simulink model "c6_pfc_rl"  (R2021b)
settings: Solver=FixedStepDiscrete  StartTime=0.0  StopTime=Inf  FixedStep=sampleTime  RelTol=1e-3  EnableMultiTasking=on
PreLoadFcn:
  | %load emptyMap
InitFcn:
  | sampleTime = 0.05;
  | nMedianSize=3;
  | 
  | % Robot parameters
  | wheelRadius = 0.0335;
  | robotRadius = 0.116;
  | 
  | % Lidar parameters
  | sensorOffset = [0,0];
  | scanAngles = linspace(-pi/2,pi/2,9)';
  | maxRange = 5;
  | 
  | %%%%%%
  | ks=1;
  | c_ks=-1;
  | 
  | 
  | 
  | 
  | 
  | 
  | % Lidar parameters
  | sensorOffset = [0,0];
  | scanAngles = linspace(-pi/3,pi/3,20)';%y = linspace(x1,x2,n) 生成 n 个点。这些点的间距为 (x2-x1)/(n-1)。
  | maxRange = 0.4;
  | 
  | %%%%%%
  | ks=1;
  | 
  | 
  | 
  | 
  | 
  | A=0.3;
  | C=1.7;
  | B=(A+C)/2;
  | 
  | wp1=[A,A; B,A;  C,A; C,B;C,C; B,C; A,C;A,B];
  | bainjie2=[-0.5,-0.5;2.5,-0.5;-0.5,2.5;2.5,2.5;]
  | WAY_P=[wp1;wp1;wp1;wp1];
  | Target=[wp1;bainjie2];
  | 
  | %%%%%%%%%%%%%%%%%%%%%%%%%%%%%%%%%%%%%%%
  | Target_robot_4=[A  A]
  | Target_robot_5=[B  A]
  | Target_robot_6=[C  A]
  | 
  | Target_robot_1=[C  C]
  | Target_robot_2=[B  C]
  | Target_robot_3=[A  C]
  | 
  | 
  | %%%%%%%%%%%%%%%%%%%%%%%%%%%%%%%%%%%%
  | 
  | 
  | 
  | 
  | 
  | % paremeters of pure persuit
  | desired_v_robot_1=0.2
  | ... (+33 lines)
undefined symbols (not defined in the file or in its folder): Angular, DiscIntNeverNeededParam, Linear
libraries: robotlib x24, dspstat3 x18, simulink x2, robotalgslib x1
(part 2 of 2)

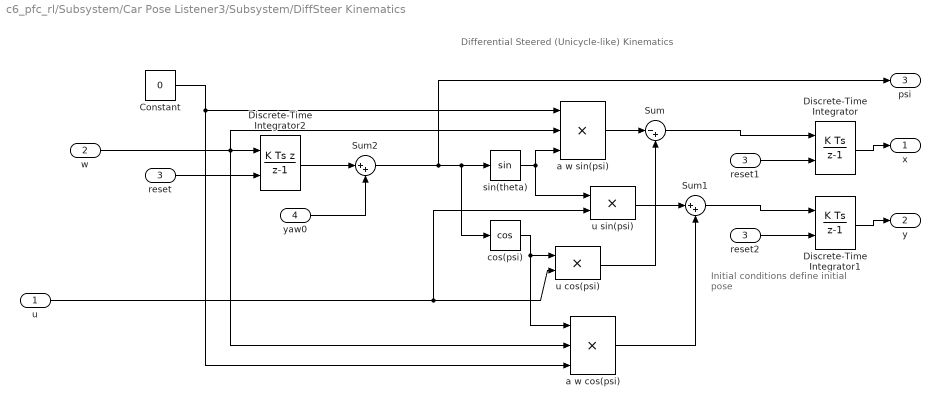
== system c6_pfc_rl/Subsystem/Car Pose Listener3/Subsystem/DiffSteer Kinematics ==
  note: Initial conditions define
      | initial pose
  note: Differential Steered (Unicycle-like) Kinematics
  u : Inport
  w : Inport  Port=2
  reset : Inport  Port=3
  yaw0 : Inport  Port=4
  Constant : Constant  Value=0
  Discrete-Time Integrator : DiscreteIntegrator  ExternalReset=falling  SampleTime=-1  ICPrevOutput=DiscIntNeverNeededParam  ICPrevScaledInput=DiscIntNeverNeededParam
  Discrete-Time Integrator1 : DiscreteIntegrator  ExternalReset=falling  SampleTime=-1  ICPrevOutput=DiscIntNeverNeededParam  ICPrevScaledInput=DiscIntNeverNeededParam
  Discrete-Time Integrator2 : DiscreteIntegrator  IntegratorMethod=Integration: Backward Euler  ExternalReset=falling  SampleTime=-1  ICPrevOutput=DiscIntNeverNeededParam  ICPrevScaledInput=DiscIntNeverNeededParam
  Sum : Sum  Inputs=|-+  SaturateOnIntegerOverflow=on
  Sum1 : Sum  Inputs=|++  SaturateOnIntegerOverflow=on
  Sum2 : Sum  Inputs=|++
  a w cos(psi) : Product  Inputs=3  SaturateOnIntegerOverflow=on  OutDataTypeStr=Inherit: Same as first input
  a w sin(psi) : Product  Inputs=3  SaturateOnIntegerOverflow=on  OutDataTypeStr=Inherit: Same as first input
  cos(psi) : Trigonometry  Operator=cos
  reset1 : InportShadow  Port=3
  reset2 : InportShadow  Port=3
  sin(theta) : Trigonometry
  u cos(psi) : Product  SaturateOnIntegerOverflow=on  OutDataTypeStr=Inherit: Same as first input
  u sin(psi) : Product  SaturateOnIntegerOverflow=on  OutDataTypeStr=Inherit: Same as first input
  x : Outport
  y : Outport  Port=2
  psi : Outport  Port=3
  wires:
  yaw0/1 -> Sum2/2
  reset2/1 -> Discrete-Time Integrator1/2
  reset1/1 -> Discrete-Time Integrator/2
  reset/1 -> Discrete-Time Integrator2/2
  u sin(psi)/1 -> Sum1/1
  cos(psi)/1 -> u cos(psi)/1, a w cos(psi)/1
  w/1 -> a w cos(psi)/2, a w sin(psi)/2, Discrete-Time Integrator2/1
  Constant/1 -> a w sin(psi)/1, a w cos(psi)/3
  Discrete-Time Integrator/1 -> x/1
  Sum/1 -> Discrete-Time Integrator/1
  sin(theta)/1 -> a w sin(psi)/3, u sin(psi)/1
  a w cos(psi)/1 -> Sum1/2
  Sum2/1 -> psi/1, sin(theta)/1, cos(psi)/1
  u cos(psi)/1 -> Sum/2
  u/1 -> u sin(psi)/2, u cos(psi)/2
  a w sin(psi)/1 -> Sum/1
  Sum1/1 -> Discrete-Time Integrator1/1
  Discrete-Time Integrator1/1 -> y/1
  Discrete-Time Integrator2/1 -> Sum2/1

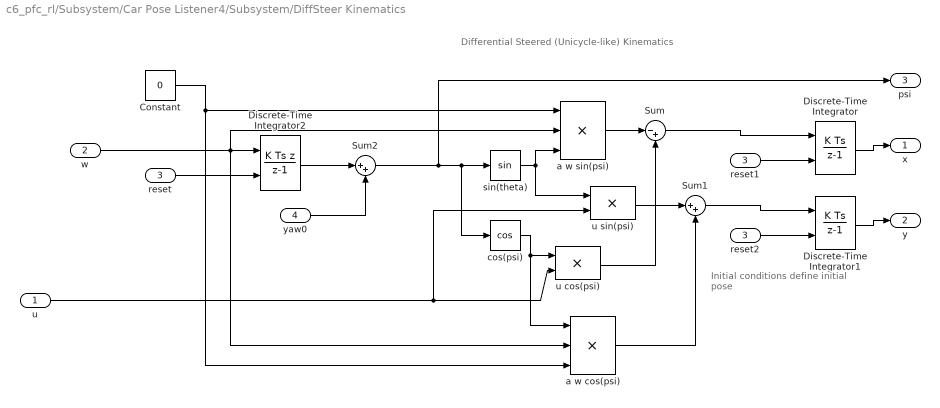
== system c6_pfc_rl/Subsystem/Car Pose Listener4/Subsystem/DiffSteer Kinematics ==
  note: Initial conditions define
      | initial pose
  note: Differential Steered (Unicycle-like) Kinematics
  u : Inport
  w : Inport  Port=2
  reset : Inport  Port=3
  yaw0 : Inport  Port=4
  Constant : Constant  Value=0
  Discrete-Time Integrator : DiscreteIntegrator  ExternalReset=falling  SampleTime=-1  ICPrevOutput=DiscIntNeverNeededParam  ICPrevScaledInput=DiscIntNeverNeededParam
  Discrete-Time Integrator1 : DiscreteIntegrator  ExternalReset=falling  SampleTime=-1  ICPrevOutput=DiscIntNeverNeededParam  ICPrevScaledInput=DiscIntNeverNeededParam
  Discrete-Time Integrator2 : DiscreteIntegrator  IntegratorMethod=Integration: Backward Euler  ExternalReset=falling  SampleTime=-1  ICPrevOutput=DiscIntNeverNeededParam  ICPrevScaledInput=DiscIntNeverNeededParam
  Sum : Sum  Inputs=|-+  SaturateOnIntegerOverflow=on
  Sum1 : Sum  Inputs=|++  SaturateOnIntegerOverflow=on
  Sum2 : Sum  Inputs=|++
  a w cos(psi) : Product  Inputs=3  SaturateOnIntegerOverflow=on  OutDataTypeStr=Inherit: Same as first input
  a w sin(psi) : Product  Inputs=3  SaturateOnIntegerOverflow=on  OutDataTypeStr=Inherit: Same as first input
  cos(psi) : Trigonometry  Operator=cos
  reset1 : InportShadow  Port=3
  reset2 : InportShadow  Port=3
  sin(theta) : Trigonometry
  u cos(psi) : Product  SaturateOnIntegerOverflow=on  OutDataTypeStr=Inherit: Same as first input
  u sin(psi) : Product  SaturateOnIntegerOverflow=on  OutDataTypeStr=Inherit: Same as first input
  x : Outport
  y : Outport  Port=2
  psi : Outport  Port=3
  wires:
  yaw0/1 -> Sum2/2
  reset2/1 -> Discrete-Time Integrator1/2
  reset1/1 -> Discrete-Time Integrator/2
  reset/1 -> Discrete-Time Integrator2/2
  u sin(psi)/1 -> Sum1/1
  cos(psi)/1 -> u cos(psi)/1, a w cos(psi)/1
  w/1 -> a w cos(psi)/2, a w sin(psi)/2, Discrete-Time Integrator2/1
  Constant/1 -> a w sin(psi)/1, a w cos(psi)/3
  Discrete-Time Integrator/1 -> x/1
  Sum/1 -> Discrete-Time Integrator/1
  sin(theta)/1 -> a w sin(psi)/3, u sin(psi)/1
  a w cos(psi)/1 -> Sum1/2
  Sum2/1 -> psi/1, sin(theta)/1, cos(psi)/1
  u cos(psi)/1 -> Sum/2
  u/1 -> u sin(psi)/2, u cos(psi)/2
  a w sin(psi)/1 -> Sum/1
  Sum1/1 -> Discrete-Time Integrator1/1
  Discrete-Time Integrator1/1 -> y/1
  Discrete-Time Integrator2/1 -> Sum2/1

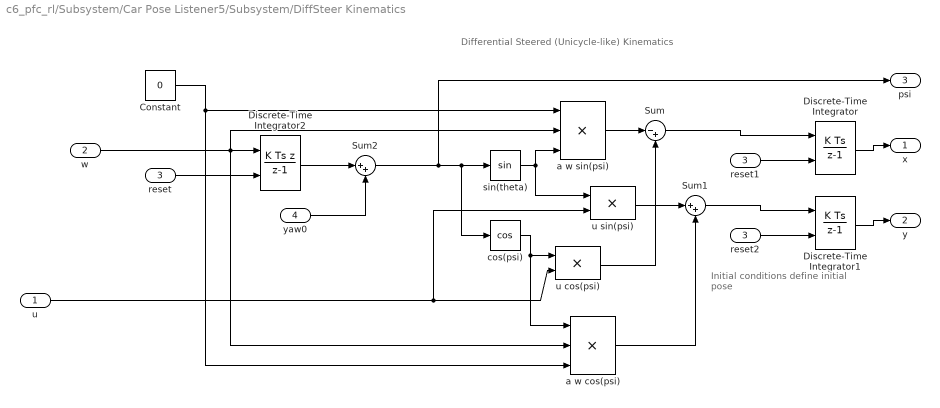
== system c6_pfc_rl/Subsystem/Car Pose Listener5/Subsystem/DiffSteer Kinematics ==
  note: Initial conditions define
      | initial pose
  note: Differential Steered (Unicycle-like) Kinematics
  u : Inport
  w : Inport  Port=2
  reset : Inport  Port=3
  yaw0 : Inport  Port=4
  Constant : Constant  Value=0
  Discrete-Time Integrator : DiscreteIntegrator  ExternalReset=falling  SampleTime=-1  ICPrevOutput=DiscIntNeverNeededParam  ICPrevScaledInput=DiscIntNeverNeededParam
  Discrete-Time Integrator1 : DiscreteIntegrator  ExternalReset=falling  SampleTime=-1  ICPrevOutput=DiscIntNeverNeededParam  ICPrevScaledInput=DiscIntNeverNeededParam
  Discrete-Time Integrator2 : DiscreteIntegrator  IntegratorMethod=Integration: Backward Euler  ExternalReset=falling  SampleTime=-1  ICPrevOutput=DiscIntNeverNeededParam  ICPrevScaledInput=DiscIntNeverNeededParam
  Sum : Sum  Inputs=|-+  SaturateOnIntegerOverflow=on
  Sum1 : Sum  Inputs=|++  SaturateOnIntegerOverflow=on
  Sum2 : Sum  Inputs=|++
  a w cos(psi) : Product  Inputs=3  SaturateOnIntegerOverflow=on  OutDataTypeStr=Inherit: Same as first input
  a w sin(psi) : Product  Inputs=3  SaturateOnIntegerOverflow=on  OutDataTypeStr=Inherit: Same as first input
  cos(psi) : Trigonometry  Operator=cos
  reset1 : InportShadow  Port=3
  reset2 : InportShadow  Port=3
  sin(theta) : Trigonometry
  u cos(psi) : Product  SaturateOnIntegerOverflow=on  OutDataTypeStr=Inherit: Same as first input
  u sin(psi) : Product  SaturateOnIntegerOverflow=on  OutDataTypeStr=Inherit: Same as first input
  x : Outport
  y : Outport  Port=2
  psi : Outport  Port=3
  wires:
  yaw0/1 -> Sum2/2
  reset2/1 -> Discrete-Time Integrator1/2
  reset1/1 -> Discrete-Time Integrator/2
  reset/1 -> Discrete-Time Integrator2/2
  u sin(psi)/1 -> Sum1/1
  cos(psi)/1 -> u cos(psi)/1, a w cos(psi)/1
  w/1 -> a w cos(psi)/2, a w sin(psi)/2, Discrete-Time Integrator2/1
  Constant/1 -> a w sin(psi)/1, a w cos(psi)/3
  Discrete-Time Integrator/1 -> x/1
  Sum/1 -> Discrete-Time Integrator/1
  sin(theta)/1 -> a w sin(psi)/3, u sin(psi)/1
  a w cos(psi)/1 -> Sum1/2
  Sum2/1 -> psi/1, sin(theta)/1, cos(psi)/1
  u cos(psi)/1 -> Sum/2
  u/1 -> u sin(psi)/2, u cos(psi)/2
  a w sin(psi)/1 -> Sum/1
  Sum1/1 -> Discrete-Time Integrator1/1
  Discrete-Time Integrator1/1 -> y/1
  Discrete-Time Integrator2/1 -> Sum2/1

== system c6_pfc_rl/controller/Subsystem1/Adjust Velocities to Avoid Obstacles/Path Following ==
  SteeringDirection : Inport
  AngularVelocity : Inport  Port=2
  Compute Angular Velocity : MATLAB Function  TreatAsAtomicUnit=on
  MaxAngularVelocity : Constant
  Subtract : Sum  Inputs=+-
  dW : Outport  VectorParamsAs1DForOutWhenUnconnected=off
  wires:
  MaxAngularVelocity/1 -> Compute Angular Velocity/2(wMax)
  SteeringDirection/1 -> Compute Angular Velocity/1(steeringDir)
  Subtract/1 -> dW/1
  Compute Angular Velocity/1(w) -> Subtract/1
  AngularVelocity/1 -> Subtract/2

== matlab function c6_pfc_rl/Subsystem/Car Pose Listener1/Subsystem/sensor2vCar ==
  data: x_init output; y_init output; yaw_init output; flag output; poseNew input; poseMsg input
function [x_init,y_init,yaw_init,flag] = sensor2vCar(poseNew, poseMsg)
persistent x0 y0 yaw0 yaw1 x0_init y0_init yaw0_init fStart
if isempty(x0)
    x0=-10; y0=-10; yaw0=0; yaw1=0;   
    x0_init=-10;y0_init=-10;yaw0_init=0;
    fStart=0;
end
if poseNew
    if x0==poseMsg.Pose.Pose.Position.X&&y0==poseMsg.Pose.Pose.Position.Y
        flag=1;
    else
        x0=poseMsg.Pose.Pose.Position.X;
        y0=poseMsg.Pose.Pose.Position.Y;   
        %yaw2=atan2(2*(poseMsg.Pose.Pose.Orientation.Z*poseMsg.Pose.Pose.Orientation.W),1-2*(poseMsg.Pose.Pose.Orientation.Z^2)); 
        eul=quat2eul([poseMsg.Pose.Pose.Orientation.W,poseMsg.Pose.Pose.Orientation.X,poseMsg.Pose.Pose.Orientation.Y,poseMsg.Pose.Pose.Orientation.Z]);
        yaw2=eul(1);
        %对前后角度差使用积分，恢复yaw的连续性
        yaw0=yaw0+angdiff(yaw1,yaw2);
        yaw1=yaw2;
        flag=0;        
        x0_init=x0;
        y0_init=y0;
        yaw0_init=yaw0;
        fStart=1;
    end 
else
    if fStart
        flag=1;
    else
        flag=0;
    end
end

x_init=x0_init;y_init=y0_init;yaw_init=yaw0_init;

== matlab function c6_pfc_rl/controller/MATLAB Function4 ==
  data: z output; pos1 input
function z = plot_a_square(pos1)
% 
% persistent Waypoints idx
% if isempty(Waypoints)
%     Waypoints=[0.2,0.2;1.8 0.2;1.8 1.8;0.2 1.8];
%     idx=0;
% end
% if idx==0
%     %初始化
%     [~,idx]=max([norm(Waypoints(1,:)-pos1(1:2)'),norm(Waypoints(2,:)-pos1(1:2)'),norm(Waypoints(3,:)-pos1(1:2)'),norm(Waypoints(4,:)-pos1(1:2)')]);
% end
% 
% if norm([Waypoints(idx,:)-pos1(1:2)'])<0.25
%     idx=idx+1;
%     if idx>length(Waypoints(:,1))
%         idx=1;
%     end
% end
% z=Waypoints(idx,:);


persistent Waypoints idx

if isempty(Waypoints)
    Waypoints=[0.5,0.5;1.5 0.5;1.5 1.5;0.5 1.5];
    idx=2;
end

if idx == 4
    pre_waypt = Waypoints(4-1,:)';
    curr_waypt = Waypoints(idx,:)';
    next_waypt = Waypoints(1,:)';
else
    if idx == 1
        pre_waypt = Waypoints(4,:)';
        curr_waypt = Waypoints(1,:)';
        next_waypt = Waypoints(2,:)';
    else
        pre_waypt = Waypoints(idx-1,:)';
        curr_waypt = Waypoints(idx,:)';
        next_waypt = Waypoints(idx+1,:)';
    end
end

pre_q = vec_norm(curr_waypt, pre_waypt);
next_q = vec_norm(next_waypt, curr_waypt);

curr_n = vec_normalize(pre_q + next_q);
curr_diff = vec_norm(pos1(1:2), curr_waypt);

flag = dot(curr_diff, curr_n);

if flag >=0

    if idx < 4
        idx = idx + 1;
    else
        idx = 1;
    end
end

idx
z=Waypoints(idx,:)

end

function result = vec_normalize(vec)
    mag = vec_mag(vec);

    if mag>0
        result = vec * (1.0/mag);
    else
        result = [0.0, 0.0];
    end
end

function result = vec_norm(vec1, vec2)
    result = vec1 - vec2;
    result = vec_normalize(result);
end

function result = vec_mag(vec)
    result = sqrt(vec(1)*vec(1)+ vec(2)*vec(2));
end

== matlab function c6_pfc_rl/controller/Ego Car Signal Process2/Signal Process ==
  data: observation output size=[1,9]; obs_flag output; pose1 input; pose2 input; leader_linear_vel input size=1; ego_linear_vel input size=1; ego_omega_vel input size=1; last_ego_omega_vel input
function [observation, obs_flag] = ...
    car2(pose1,pose2,leader_linear_vel, ego_linear_vel, ego_omega_vel, last_ego_omega_vel)


persistent sim_step  yaw_delta lateral_rel_dist

if isempty(sim_step)
    sim_step = 0;
end

if isempty(yaw_delta)
    yaw_delta = 0.0;
end

if isempty(lateral_rel_dist)
    lateral_rel_dist = 0.0;
end

x1=pose1(1);
y1=pose1(2);
yaw1=pose1(3);

x2=pose2(1);
y2=pose2(2);
yaw2=pose2(3);
obs_flag = 1;
observation = zeros(1,9);

if isnan(yaw1)||isnan(yaw2)
    observation = zeros(1,9);
    obs_flag = 0;
    yaw_delta_new = 0.0;
    lateral_rel_dist_new = 0.0;
else
    yaw_delta_new = angdiff(yaw1, yaw2);
    
    [~, lateral_rel_dist_new, longitudinal_rel_dist_new] = heng_zong_dist_calc(x1,y1,x2,y2, yaw1);
    
    observation = get_obs(x1,x2,y1,y2,lateral_rel_dist_new, longitudinal_rel_dist_new, ...
        yaw_delta_new, leader_linear_vel, ego_linear_vel, yaw_delta, lateral_rel_dist); 
end

sim_step = sim_step + 1;
yaw_delta = yaw_delta_new;
lateral_rel_dist = lateral_rel_dist_new;

end

function [rel_dist, heng_dist, zong_dist] = heng_zong_dist_calc(x1,y1,x2,y2, yaw1)

rel_yaw = atan2(y2-y1, x2-x1);

yaw_delta = angdiff(yaw1, rel_yaw);

rel_dist = sqrt(power(x2-x1,2.0)+power(y2-y1,2.0));

heng_dist = rel_dist*sin(yaw_delta);

zong_dist = rel_dist*cos(yaw_delta);

end

function v_ref = get_ref_velocity(leader_linear_vel, ego_linear_vel, longitudinal_rel_dist)
    t_gap = 1.0;
    D_default = 0.3;
    ego_v_set = 0.2;
    d_safe = ego_linear_vel * t_gap + D_default;

    if d_safe > longitudinal_rel_dist
        v_ref = min(leader_linear_vel, ego_v_set);
    else
        v_ref = ego_v_set;
    end
end

function observation = get_obs(x1,x2,y1,y2,lateral_rel_dist_new, longitudinal_rel_dist_new, ...
    yaw_delta_new, leader_linear_vel, ego_linear_vel, yaw_delta, lateral_rel_dist)  
    % 状态空间
    % longitudinal_rel_dist 前车与后车的纵向相对距离
    % lateral_rel_dist 前车与后车的横向相对距离
    % yaw_delta 前车与后车的航向角偏差
    % ego_linear_vel 后车的线速度
    % e_v 后车的参考速度与线速度之差
    % lateral_rel_dist_dot 前车与后车的横向相对距离变化率
    % yaw_delta_dot 前车与后车的航向角偏差变化率

    % 计算前车与后车的相对位置
    x_delta = x1 - x2;
    y_delta = y1 - y2;
    
    % 计算后车的横向偏移距离变化率和相对航向角变化率
    lateral_rel_dist_dot = lateral_rel_dist_new - lateral_rel_dist;
    yaw_delta_dot = yaw_delta_new - yaw_delta;

    % 计算后车的参考速度与线速度之差
    v_ref = get_ref_velocity(leader_linear_vel, ego_linear_vel, longitudinal_rel_dist_new);
    e_v = v_ref - ego_linear_vel;

    observation = [x_delta/2.0, y_delta/2.0, longitudinal_rel_dist_new/2.0, e_v/0.5, ego_linear_vel/0.5, ...
        lateral_rel_dist_new/2.0, lateral_rel_dist_dot/2.0, yaw_delta_new/pi, yaw_delta_dot/pi];
end

function flag = EnvisDone(rel_dist, lateral_rel_dist, longitudinal_rel_dist)
    flag = 0;
    avoid_dist = 0.14;

    max_lateral_rel_dist= 0.45;
    min_longitudinal_rel_dist = -0.5;

    if rel_dist <= avoid_dist
        flag = 1;
    end

    if longitudinal_rel_dist <= min_longitudinal_rel_dist
        flag = 1;
    end
    
    if abs(lateral_rel_dist) >= max_lateral_rel_dist
        flag = 1;
    end
end

function reward = reward_calc(e_v, lateral_rel_dist, ego_linear_vel, ego_omega_vel, last_ego_omega_vel, isDone, sim_step)
    F_t = 0.0;
    M_t = 0.0;
    H_t = 0.0;
    delta_omega = 0.0;
    
    e_v_square = e_v * e_v;
    lateral_rel_dist_square = lateral_rel_dist * lateral_rel_dist;

    if isDone==1
        F_t = 1.0;
    end

    if e_v_square < 1.0
        M_t = 1.0;
    end

    if lateral_rel_dist_square<0.01
        H_t = 1.0;
    end

    if sim_step >= 2
        delta_omega = ego_omega_vel - last_ego_omega_vel;
    end

    reward = -0.1*e_v_square - 0.1*ego_linear_vel*ego_linear_vel -0.1*lateral_rel_dist_square ...
         - 0.5*ego_omega_vel*ego_omega_vel -0.4*delta_omega*delta_omega - 10.0*F_t + M_t + + 2.0*H_t;

end

== matlab function c6_pfc_rl/Subsystem/Car Pose Listener/Subsystem/sensor2vCar4 ==
  data: V output; W output; VW_New input; VW_Msg input
function [V,W] = sensor2vCar(VW_New, VW_Msg)
persistent v0 w0
if isempty(v0)
    v0=0; 
    w0=0;    
end
if VW_New
    v0=VW_Msg.Linear.X;
    w0=VW_Msg.Angular.Z;
end

V=v0;
W=-w0;

== matlab function c6_pfc_rl/controller/MATLAB Function2 ==
  settings: updateMethod=DISCRETE
  data: obs input double size=9; pose2 input; action output double size=[1,2]; obs_flag input
function action = one_car_pfc(obs, pose2, obs_flag)

longitudinal_rel_dist = obs(3);
lateral_rel_dist = obs(6);

if longitudinal_rel_dist > -0.25 && abs(lateral_rel_dist) <=0.225 && longitudinal_rel_dist < 0
    action = double(PFC_Policy(obs));
else
    action = simple_pfc(obs(1), obs(2), pose2(3));
end

if obs_flag==0
    action = [0.0, 0.0];
end

end

function action = simple_pfc(x_delta, y_delta, yaw2)
    kk = -1.0;

    new_theta_cmd = atan2(y_delta, x_delta);
    
    delta_theta = angdiff(yaw2, new_theta_cmd);

    angular_speed = kk * delta_theta;
     
    new_omega_cmd = angular_speed;

    action = [0.225, new_omega_cmd];

end

== matlab function c6_pfc_rl/controller/Ego Car Signal Process3/Signal Process ==
  data: observation output size=[1,9]; obs_flag output; pose1 input; pose2 input; leader_linear_vel input size=1; ego_linear_vel input size=1; ego_omega_vel input size=1; last_ego_omega_vel input
function [observation, obs_flag] = ...
    car2(pose1,pose2,leader_linear_vel, ego_linear_vel, ego_omega_vel, last_ego_omega_vel)


persistent sim_step  yaw_delta lateral_rel_dist

if isempty(sim_step)
    sim_step = 0;
end

if isempty(yaw_delta)
    yaw_delta = 0.0;
end

if isempty(lateral_rel_dist)
    lateral_rel_dist = 0.0;
end

x1=pose1(1);
y1=pose1(2);
yaw1=pose1(3);

x2=pose2(1);
y2=pose2(2);
yaw2=pose2(3);
obs_flag = 1;
observation = zeros(1,9);

if isnan(yaw1)||isnan(yaw2)
    observation = zeros(1,9);
    obs_flag = 0;
    yaw_delta_new = 0.0;
    lateral_rel_dist_new = 0.0;
else
    yaw_delta_new = angdiff(yaw1, yaw2);
    
    [~, lateral_rel_dist_new, longitudinal_rel_dist_new] = heng_zong_dist_calc(x1,y1,x2,y2, yaw1);
    
    observation = get_obs(x1,x2,y1,y2,lateral_rel_dist_new, longitudinal_rel_dist_new, ...
        yaw_delta_new, leader_linear_vel, ego_linear_vel, yaw_delta, lateral_rel_dist); 
end

sim_step = sim_step + 1;
yaw_delta = yaw_delta_new;
lateral_rel_dist = lateral_rel_dist_new;

end

function [rel_dist, heng_dist, zong_dist] = heng_zong_dist_calc(x1,y1,x2,y2, yaw1)

rel_yaw = atan2(y2-y1, x2-x1);

yaw_delta = angdiff(yaw1, rel_yaw);

rel_dist = sqrt(power(x2-x1,2.0)+power(y2-y1,2.0));

heng_dist = rel_dist*sin(yaw_delta);

zong_dist = rel_dist*cos(yaw_delta);

end

function v_ref = get_ref_velocity(leader_linear_vel, ego_linear_vel, longitudinal_rel_dist)
    t_gap = 1.0;
    D_default = 0.3;
    ego_v_set = 0.2;
    d_safe = ego_linear_vel * t_gap + D_default;

    if d_safe > longitudinal_rel_dist
        v_ref = min(leader_linear_vel, ego_v_set);
    else
        v_ref = ego_v_set;
    end
end

function observation = get_obs(x1,x2,y1,y2,lateral_rel_dist_new, longitudinal_rel_dist_new, ...
    yaw_delta_new, leader_linear_vel, ego_linear_vel, yaw_delta, lateral_rel_dist)  
    % 状态空间
    % longitudinal_rel_dist 前车与后车的纵向相对距离
    % lateral_rel_dist 前车与后车的横向相对距离
    % yaw_delta 前车与后车的航向角偏差
    % ego_linear_vel 后车的线速度
    % e_v 后车的参考速度与线速度之差
    % lateral_rel_dist_dot 前车与后车的横向相对距离变化率
    % yaw_delta_dot 前车与后车的航向角偏差变化率

    % 计算前车与后车的相对位置
    x_delta = x1 - x2;
    y_delta = y1 - y2;
    
    % 计算后车的横向偏移距离变化率和相对航向角变化率
    lateral_rel_dist_dot = lateral_rel_dist_new - lateral_rel_dist;
    yaw_delta_dot = yaw_delta_new - yaw_delta;

    % 计算后车的参考速度与线速度之差
    v_ref = get_ref_velocity(leader_linear_vel, ego_linear_vel, longitudinal_rel_dist_new);
    e_v = v_ref - ego_linear_vel;

    observation = [x_delta/2.0, y_delta/2.0, longitudinal_rel_dist_new/2.0, e_v/0.5, ego_linear_vel/0.5, ...
        lateral_rel_dist_new/2.0, lateral_rel_dist_dot/2.0, yaw_delta_new/pi, yaw_delta_dot/pi];
end

function flag = EnvisDone(rel_dist, lateral_rel_dist, longitudinal_rel_dist)
    flag = 0;
    avoid_dist = 0.14;

    max_lateral_rel_dist= 0.45;
    min_longitudinal_rel_dist = -0.5;

    if rel_dist <= avoid_dist
        flag = 1;
    end

    if longitudinal_rel_dist <= min_longitudinal_rel_dist
        flag = 1;
    end
    
    if abs(lateral_rel_dist) >= max_lateral_rel_dist
        flag = 1;
    end
end

function reward = reward_calc(e_v, lateral_rel_dist, ego_linear_vel, ego_omega_vel, last_ego_omega_vel, isDone, sim_step)
    F_t = 0.0;
    M_t = 0.0;
    H_t = 0.0;
    delta_omega = 0.0;
    
    e_v_square = e_v * e_v;
    lateral_rel_dist_square = lateral_rel_dist * lateral_rel_dist;

    if isDone==1
        F_t = 1.0;
    end

    if e_v_square < 1.0
        M_t = 1.0;
    end

    if lateral_rel_dist_square<0.01
        H_t = 1.0;
    end

    if sim_step >= 2
        delta_omega = ego_omega_vel - last_ego_omega_vel;
    end

    reward = -0.1*e_v_square - 0.1*ego_linear_vel*ego_linear_vel -0.1*lateral_rel_dist_square ...
         - 0.5*ego_omega_vel*ego_omega_vel -0.4*delta_omega*delta_omega - 10.0*F_t + M_t + + 2.0*H_t;

end

== matlab function c6_pfc_rl/controller/MATLAB Function3 ==
  settings: updateMethod=DISCRETE
  data: obs input double size=9; pose2 input; action output double size=[1,2]; obs_flag input
function action = one_car_pfc(obs, pose2, obs_flag)

longitudinal_rel_dist = obs(3);
lateral_rel_dist = obs(6);

if longitudinal_rel_dist > -0.25 && abs(lateral_rel_dist) <=0.225 && longitudinal_rel_dist < 0
    action = double(PFC_Policy(obs));
else
    action = simple_pfc(obs(1), obs(2), pose2(3));
end

if obs_flag==0
    action = [0.0, 0.0];
end

end

function action = simple_pfc(x_delta, y_delta, yaw2)
    kk = -1.0;

    new_theta_cmd = atan2(y_delta, x_delta);
    
    delta_theta = angdiff(yaw2, new_theta_cmd);

    angular_speed = kk * delta_theta;
     
    new_omega_cmd = angular_speed;

    action = [0.225*1.2, new_omega_cmd];

end

== matlab function c6_pfc_rl/controller/MATLAB Function5 ==
  settings: updateMethod=DISCRETE
  data: obs input double size=9; pose2 input; action output double size=[1,2]; obs_flag input
function action = one_car_pfc(obs, pose2, obs_flag)

longitudinal_rel_dist = obs(3);
lateral_rel_dist = obs(6);

if longitudinal_rel_dist > -0.25 && abs(lateral_rel_dist) <=0.225 && longitudinal_rel_dist < 0
    action = double(PFC_Policy(obs));
else
    action = simple_pfc(obs(1), obs(2), pose2(3));
end

if obs_flag==0
    action = [0.0, 0.0];
end

end

function action = simple_pfc(x_delta, y_delta, yaw2)
    kk = -1.0;

    new_theta_cmd = atan2(y_delta, x_delta);
    
    delta_theta = angdiff(yaw2, new_theta_cmd);

    angular_speed = kk * delta_theta;
     
    new_omega_cmd = angular_speed;

    action = [0.225*1.5, new_omega_cmd];

end

== matlab function c6_pfc_rl/controller/Ego Car Signal Process4/Signal Process ==
  data: observation output size=[1,9]; obs_flag output; pose1 input; pose2 input; leader_linear_vel input size=1; ego_linear_vel input size=1; ego_omega_vel input size=1; last_ego_omega_vel input
function [observation, obs_flag] = ...
    car2(pose1,pose2,leader_linear_vel, ego_linear_vel, ego_omega_vel, last_ego_omega_vel)


persistent sim_step  yaw_delta lateral_rel_dist

if isempty(sim_step)
    sim_step = 0;
end

if isempty(yaw_delta)
    yaw_delta = 0.0;
end

if isempty(lateral_rel_dist)
    lateral_rel_dist = 0.0;
end

x1=pose1(1);
y1=pose1(2);
yaw1=pose1(3);

x2=pose2(1);
y2=pose2(2);
yaw2=pose2(3);
obs_flag = 1;
observation = zeros(1,9);

if isnan(yaw1)||isnan(yaw2)
    observation = zeros(1,9);
    obs_flag = 0;
    yaw_delta_new = 0.0;
    lateral_rel_dist_new = 0.0;
else
    yaw_delta_new = angdiff(yaw1, yaw2);
    
    [~, lateral_rel_dist_new, longitudinal_rel_dist_new] = heng_zong_dist_calc(x1,y1,x2,y2, yaw1);
    
    observation = get_obs(x1,x2,y1,y2,lateral_rel_dist_new, longitudinal_rel_dist_new, ...
        yaw_delta_new, leader_linear_vel, ego_linear_vel, yaw_delta, lateral_rel_dist); 
end

sim_step = sim_step + 1;
yaw_delta = yaw_delta_new;
lateral_rel_dist = lateral_rel_dist_new;

end

function [rel_dist, heng_dist, zong_dist] = heng_zong_dist_calc(x1,y1,x2,y2, yaw1)

rel_yaw = atan2(y2-y1, x2-x1);

yaw_delta = angdiff(yaw1, rel_yaw);

rel_dist = sqrt(power(x2-x1,2.0)+power(y2-y1,2.0));

heng_dist = rel_dist*sin(yaw_delta);

zong_dist = rel_dist*cos(yaw_delta);

end

function v_ref = get_ref_velocity(leader_linear_vel, ego_linear_vel, longitudinal_rel_dist)
    t_gap = 1.0;
    D_default = 0.3;
    ego_v_set = 0.2;
    d_safe = ego_linear_vel * t_gap + D_default;

    if d_safe > longitudinal_rel_dist
        v_ref = min(leader_linear_vel, ego_v_set);
    else
        v_ref = ego_v_set;
    end
end

function observation = get_obs(x1,x2,y1,y2,lateral_rel_dist_new, longitudinal_rel_dist_new, ...
    yaw_delta_new, leader_linear_vel, ego_linear_vel, yaw_delta, lateral_rel_dist)  
    % 状态空间
    % longitudinal_rel_dist 前车与后车的纵向相对距离
    % lateral_rel_dist 前车与后车的横向相对距离
    % yaw_delta 前车与后车的航向角偏差
    % ego_linear_vel 后车的线速度
    % e_v 后车的参考速度与线速度之差
    % lateral_rel_dist_dot 前车与后车的横向相对距离变化率
    % yaw_delta_dot 前车与后车的航向角偏差变化率

    % 计算前车与后车的相对位置
    x_delta = x1 - x2;
    y_delta = y1 - y2;
    
    % 计算后车的横向偏移距离变化率和相对航向角变化率
    lateral_rel_dist_dot = lateral_rel_dist_new - lateral_rel_dist;
    yaw_delta_dot = yaw_delta_new - yaw_delta;

    % 计算后车的参考速度与线速度之差
    v_ref = get_ref_velocity(leader_linear_vel, ego_linear_vel, longitudinal_rel_dist_new);
    e_v = v_ref - ego_linear_vel;

    observation = [x_delta/2.0, y_delta/2.0, longitudinal_rel_dist_new/2.0, e_v/0.5, ego_linear_vel/0.5, ...
        lateral_rel_dist_new/2.0, lateral_rel_dist_dot/2.0, yaw_delta_new/pi, yaw_delta_dot/pi];
end

function flag = EnvisDone(rel_dist, lateral_rel_dist, longitudinal_rel_dist)
    flag = 0;
    avoid_dist = 0.14;

    max_lateral_rel_dist= 0.45;
    min_longitudinal_rel_dist = -0.5;

    if rel_dist <= avoid_dist
        flag = 1;
    end

    if longitudinal_rel_dist <= min_longitudinal_rel_dist
        flag = 1;
    end
    
    if abs(lateral_rel_dist) >= max_lateral_rel_dist
        flag = 1;
    end
end

function reward = reward_calc(e_v, lateral_rel_dist, ego_linear_vel, ego_omega_vel, last_ego_omega_vel, isDone, sim_step)
    F_t = 0.0;
    M_t = 0.0;
    H_t = 0.0;
    delta_omega = 0.0;
    
    e_v_square = e_v * e_v;
    lateral_rel_dist_square = lateral_rel_dist * lateral_rel_dist;

    if isDone==1
        F_t = 1.0;
    end

    if e_v_square < 1.0
        M_t = 1.0;
    end

    if lateral_rel_dist_square<0.01
        H_t = 1.0;
    end

    if sim_step >= 2
        delta_omega = ego_omega_vel - last_ego_omega_vel;
    end

    reward = -0.1*e_v_square - 0.1*ego_linear_vel*ego_linear_vel -0.1*lateral_rel_dist_square ...
         - 0.5*ego_omega_vel*ego_omega_vel -0.4*delta_omega*delta_omega - 10.0*F_t + M_t + + 2.0*H_t;

end

== matlab function c6_pfc_rl/controller/MATLAB Function6 ==
  settings: updateMethod=DISCRETE
  data: obs input double size=9; pose2 input; action output double size=[1,2]; obs_flag input
function action = one_car_pfc(obs, pose2, obs_flag)

longitudinal_rel_dist = obs(3);
lateral_rel_dist = obs(6);

if longitudinal_rel_dist > -0.25 && abs(lateral_rel_dist) <=0.225 && longitudinal_rel_dist < 0
    action = double(PFC_Policy(obs));
else
    action = simple_pfc(obs(1), obs(2), pose2(3));
end

if obs_flag==0
    action = [0.0, 0.0];
end

end

function action = simple_pfc(x_delta, y_delta, yaw2)
    kk = -1.0;

    new_theta_cmd = atan2(y_delta, x_delta);
    
    delta_theta = angdiff(yaw2, new_theta_cmd);

    angular_speed = kk * delta_theta;
     
    new_omega_cmd = angular_speed;

    action = [0.225, new_omega_cmd];

end

== matlab function c6_pfc_rl/Subsystem/Car Pose Listener3/Subsystem/sensor2vCar ==
  data: x_init output; y_init output; yaw_init output; flag output; poseNew input; poseMsg input
function [x_init,y_init,yaw_init,flag] = sensor2vCar(poseNew, poseMsg)
persistent x0 y0 yaw0 yaw1 x0_init y0_init yaw0_init fStart
if isempty(x0)
    x0=-10; y0=-10; yaw0=0; yaw1=0;   
    x0_init=-10;y0_init=-10;yaw0_init=0;
    fStart=0;
end
if poseNew
    if x0==poseMsg.Pose.Pose.Position.X&&y0==poseMsg.Pose.Pose.Position.Y
        flag=1;
    else
        x0=poseMsg.Pose.Pose.Position.X;
        y0=poseMsg.Pose.Pose.Position.Y;   
        %yaw2=atan2(2*(poseMsg.Pose.Pose.Orientation.Z*poseMsg.Pose.Pose.Orientation.W),1-2*(poseMsg.Pose.Pose.Orientation.Z^2)); 
        eul=quat2eul([poseMsg.Pose.Pose.Orientation.W,poseMsg.Pose.Pose.Orientation.X,poseMsg.Pose.Pose.Orientation.Y,poseMsg.Pose.Pose.Orientation.Z]);
        yaw2=eul(1);
        %对前后角度差使用积分，恢复yaw的连续性
        yaw0=yaw0+angdiff(yaw1,yaw2);
        yaw1=yaw2;
        flag=0;        
        x0_init=x0;
        y0_init=y0;
        yaw0_init=yaw0;
        fStart=1;
    end 
else
    if fStart
        flag=1;
    else
        flag=0;
    end
end

x_init=x0_init;y_init=y0_init;yaw_init=yaw0_init;

== matlab function c6_pfc_rl/controller/Ego Car Signal Process5/Signal Process ==
  data: observation output size=[1,9]; obs_flag output; pose1 input; pose2 input; leader_linear_vel input size=1; ego_linear_vel input size=1; ego_omega_vel input size=1; last_ego_omega_vel input
function [observation, obs_flag] = ...
    car2(pose1,pose2,leader_linear_vel, ego_linear_vel, ego_omega_vel, last_ego_omega_vel)


persistent sim_step  yaw_delta lateral_rel_dist

if isempty(sim_step)
    sim_step = 0;
end

if isempty(yaw_delta)
    yaw_delta = 0.0;
end

if isempty(lateral_rel_dist)
    lateral_rel_dist = 0.0;
end

x1=pose1(1);
y1=pose1(2);
yaw1=pose1(3);

x2=pose2(1);
y2=pose2(2);
yaw2=pose2(3);
obs_flag = 1;
observation = zeros(1,9);

if isnan(yaw1)||isnan(yaw2)
    observation = zeros(1,9);
    obs_flag = 0;
    yaw_delta_new = 0.0;
    lateral_rel_dist_new = 0.0;
else
    yaw_delta_new = angdiff(yaw1, yaw2);
    
    [~, lateral_rel_dist_new, longitudinal_rel_dist_new] = heng_zong_dist_calc(x1,y1,x2,y2, yaw1);
    
    observation = get_obs(x1,x2,y1,y2,lateral_rel_dist_new, longitudinal_rel_dist_new, ...
        yaw_delta_new, leader_linear_vel, ego_linear_vel, yaw_delta, lateral_rel_dist); 
end

sim_step = sim_step + 1;
yaw_delta = yaw_delta_new;
lateral_rel_dist = lateral_rel_dist_new;

end

function [rel_dist, heng_dist, zong_dist] = heng_zong_dist_calc(x1,y1,x2,y2, yaw1)

rel_yaw = atan2(y2-y1, x2-x1);

yaw_delta = angdiff(yaw1, rel_yaw);

rel_dist = sqrt(power(x2-x1,2.0)+power(y2-y1,2.0));

heng_dist = rel_dist*sin(yaw_delta);

zong_dist = rel_dist*cos(yaw_delta);

end

function v_ref = get_ref_velocity(leader_linear_vel, ego_linear_vel, longitudinal_rel_dist)
    t_gap = 1.0;
    D_default = 0.3;
    ego_v_set = 0.2;
    d_safe = ego_linear_vel * t_gap + D_default;

    if d_safe > longitudinal_rel_dist
        v_ref = min(leader_linear_vel, ego_v_set);
    else
        v_ref = ego_v_set;
    end
end

function observation = get_obs(x1,x2,y1,y2,lateral_rel_dist_new, longitudinal_rel_dist_new, ...
    yaw_delta_new, leader_linear_vel, ego_linear_vel, yaw_delta, lateral_rel_dist)  
    % 状态空间
    % longitudinal_rel_dist 前车与后车的纵向相对距离
    % lateral_rel_dist 前车与后车的横向相对距离
    % yaw_delta 前车与后车的航向角偏差
    % ego_linear_vel 后车的线速度
    % e_v 后车的参考速度与线速度之差
    % lateral_rel_dist_dot 前车与后车的横向相对距离变化率
    % yaw_delta_dot 前车与后车的航向角偏差变化率

    % 计算前车与后车的相对位置
    x_delta = x1 - x2;
    y_delta = y1 - y2;
    
    % 计算后车的横向偏移距离变化率和相对航向角变化率
    lateral_rel_dist_dot = lateral_rel_dist_new - lateral_rel_dist;
    yaw_delta_dot = yaw_delta_new - yaw_delta;

    % 计算后车的参考速度与线速度之差
    v_ref = get_ref_velocity(leader_linear_vel, ego_linear_vel, longitudinal_rel_dist_new);
    e_v = v_ref - ego_linear_vel;

    observation = [x_delta/2.0, y_delta/2.0, longitudinal_rel_dist_new/2.0, e_v/0.5, ego_linear_vel/0.5, ...
        lateral_rel_dist_new/2.0, lateral_rel_dist_dot/2.0, yaw_delta_new/pi, yaw_delta_dot/pi];
end

function flag = EnvisDone(rel_dist, lateral_rel_dist, longitudinal_rel_dist)
    flag = 0;
    avoid_dist = 0.14;

    max_lateral_rel_dist= 0.45;
    min_longitudinal_rel_dist = -0.5;

    if rel_dist <= avoid_dist
        flag = 1;
    end

    if longitudinal_rel_dist <= min_longitudinal_rel_dist
        flag = 1;
    end
    
    if abs(lateral_rel_dist) >= max_lateral_rel_dist
        flag = 1;
    end
end

function reward = reward_calc(e_v, lateral_rel_dist, ego_linear_vel, ego_omega_vel, last_ego_omega_vel, isDone, sim_step)
    F_t = 0.0;
    M_t = 0.0;
    H_t = 0.0;
    delta_omega = 0.0;
    
    e_v_square = e_v * e_v;
    lateral_rel_dist_square = lateral_rel_dist * lateral_rel_dist;

    if isDone==1
        F_t = 1.0;
    end

    if e_v_square < 1.0
        M_t = 1.0;
    end

    if lateral_rel_dist_square<0.01
        H_t = 1.0;
    end

    if sim_step >= 2
        delta_omega = ego_omega_vel - last_ego_omega_vel;
    end

    reward = -0.1*e_v_square - 0.1*ego_linear_vel*ego_linear_vel -0.1*lateral_rel_dist_square ...
         - 0.5*ego_omega_vel*ego_omega_vel -0.4*delta_omega*delta_omega - 10.0*F_t + M_t + + 2.0*H_t;

end

== matlab function c6_pfc_rl/Subsystem/Car Pose Listener3/Subsystem/sensor2vCar4 ==
  data: V output; W output; VW_New input; VW_Msg input
function [V,W] = sensor2vCar(VW_New, VW_Msg)
persistent v0 w0
if isempty(v0)
    v0=0; 
    w0=0;    
end
if VW_New
    v0=VW_Msg.Linear.X;
    w0=VW_Msg.Angular.Z;
end

V=v0;
W=-w0;

== matlab function c6_pfc_rl/Subsystem/Car Pose Listener4/Subsystem/sensor2vCar ==
  data: x_init output; y_init output; yaw_init output; flag output; poseNew input; poseMsg input
function [x_init,y_init,yaw_init,flag] = sensor2vCar(poseNew, poseMsg)
persistent x0 y0 yaw0 yaw1 x0_init y0_init yaw0_init fStart
if isempty(x0)
    x0=-10; y0=-10; yaw0=0; yaw1=0;   
    x0_init=-10;y0_init=-10;yaw0_init=0;
    fStart=0;
end
if poseNew
    if x0==poseMsg.Pose.Pose.Position.X&&y0==poseMsg.Pose.Pose.Position.Y
        flag=1;
    else
        x0=poseMsg.Pose.Pose.Position.X;
        y0=poseMsg.Pose.Pose.Position.Y;   
        %yaw2=atan2(2*(poseMsg.Pose.Pose.Orientation.Z*poseMsg.Pose.Pose.Orientation.W),1-2*(poseMsg.Pose.Pose.Orientation.Z^2)); 
        eul=quat2eul([poseMsg.Pose.Pose.Orientation.W,poseMsg.Pose.Pose.Orientation.X,poseMsg.Pose.Pose.Orientation.Y,poseMsg.Pose.Pose.Orientation.Z]);
        yaw2=eul(1);
        %对前后角度差使用积分，恢复yaw的连续性
        yaw0=yaw0+angdiff(yaw1,yaw2);
        yaw1=yaw2;
        flag=0;        
        x0_init=x0;
        y0_init=y0;
        yaw0_init=yaw0;
        fStart=1;
    end 
else
    if fStart
        flag=1;
    else
        flag=0;
    end
end

x_init=x0_init;y_init=y0_init;yaw_init=yaw0_init;

== matlab function c6_pfc_rl/Subsystem/Car Pose Listener4/Subsystem/sensor2vCar4 ==
  data: V output; W output; VW_New input; VW_Msg input
function [V,W] = sensor2vCar(VW_New, VW_Msg)
persistent v0 w0
if isempty(v0)
    v0=0; 
    w0=0;    
end
if VW_New
    v0=VW_Msg.Linear.X;
    w0=VW_Msg.Angular.Z;
end

V=v0;
W=-w0;

== matlab function c6_pfc_rl/Subsystem/Car Pose Listener5/Subsystem/sensor2vCar ==
  data: x_init output; y_init output; yaw_init output; flag output; poseNew input; poseMsg input
function [x_init,y_init,yaw_init,flag] = sensor2vCar(poseNew, poseMsg)
persistent x0 y0 yaw0 yaw1 x0_init y0_init yaw0_init fStart
if isempty(x0)
    x0=-10; y0=-10; yaw0=0; yaw1=0;   
    x0_init=-10;y0_init=-10;yaw0_init=0;
    fStart=0;
end
if poseNew
    if x0==poseMsg.Pose.Pose.Position.X&&y0==poseMsg.Pose.Pose.Position.Y
        flag=1;
    else
        x0=poseMsg.Pose.Pose.Position.X;
        y0=poseMsg.Pose.Pose.Position.Y;   
        %yaw2=atan2(2*(poseMsg.Pose.Pose.Orientation.Z*poseMsg.Pose.Pose.Orientation.W),1-2*(poseMsg.Pose.Pose.Orientation.Z^2)); 
        eul=quat2eul([poseMsg.Pose.Pose.Orientation.W,poseMsg.Pose.Pose.Orientation.X,poseMsg.Pose.Pose.Orientation.Y,poseMsg.Pose.Pose.Orientation.Z]);
        yaw2=eul(1);
        %对前后角度差使用积分，恢复yaw的连续性
        yaw0=yaw0+angdiff(yaw1,yaw2);
        yaw1=yaw2;
        flag=0;        
        x0_init=x0;
        y0_init=y0;
        yaw0_init=yaw0;
        fStart=1;
    end 
else
    if fStart
        flag=1;
    else
        flag=0;
    end
end

x_init=x0_init;y_init=y0_init;yaw_init=yaw0_init;

== matlab function c6_pfc_rl/Subsystem/Car Pose Listener5/Subsystem/sensor2vCar4 ==
  data: V output; W output; VW_New input; VW_Msg input
function [V,W] = sensor2vCar(VW_New, VW_Msg)
persistent v0 w0
if isempty(v0)
    v0=0; 
    w0=0;    
end
if VW_New
    v0=VW_Msg.Linear.X;
    w0=VW_Msg.Angular.Z;
end

V=v0;
W=-w0;

== matlab function c6_pfc_rl/Subsystem/Car Pose Listener/Subsystem/sensor2vCar ==
  data: x_init output; y_init output; yaw_init output; flag output; poseNew input; poseMsg input
function [x_init,y_init,yaw_init,flag] = sensor2vCar(poseNew, poseMsg)
persistent x0 y0 yaw0 yaw1 x0_init y0_init yaw0_init fStart
if isempty(x0)
    x0=-10; y0=-10; yaw0=0; yaw1=0;   
    x0_init=-10;y0_init=-10;yaw0_init=0;
    fStart=0;
end
if poseNew
    if x0==poseMsg.Pose.Pose.Position.X&&y0==poseMsg.Pose.Pose.Position.Y
        flag=1;
    else
        x0=poseMsg.Pose.Pose.Position.X;
        y0=poseMsg.Pose.Pose.Position.Y;   
        %yaw2=atan2(2*(poseMsg.Pose.Pose.Orientation.Z*poseMsg.Pose.Pose.Orientation.W),1-2*(poseMsg.Pose.Pose.Orientation.Z^2)); 
        eul=quat2eul([poseMsg.Pose.Pose.Orientation.W,poseMsg.Pose.Pose.Orientation.X,poseMsg.Pose.Pose.Orientation.Y,poseMsg.Pose.Pose.Orientation.Z]);
        yaw2=eul(1);
        %对前后角度差使用积分，恢复yaw的连续性
        yaw0=yaw0+angdiff(yaw1,yaw2);
        yaw1=yaw2;
        flag=0;        
        x0_init=x0;
        y0_init=y0;
        yaw0_init=yaw0;
        fStart=1;
    end 
else
    if fStart
        flag=1;
    else
        flag=0;
    end
end

x_init=x0_init;y_init=y0_init;yaw_init=yaw0_init;

== matlab function c6_pfc_rl/Subsystem/Car Pose Listener1/Subsystem/sensor2vCar4 ==
  data: V output; W output; VW_New input; VW_Msg input
function [V,W] = sensor2vCar(VW_New, VW_Msg)
persistent v0 w0
if isempty(v0)
    v0=0; 
    w0=0;    
end
if VW_New
    v0=VW_Msg.Linear.X;
    w0=VW_Msg.Angular.Z;
end

V=v0;
W=-w0;

== matlab function c6_pfc_rl/Subsystem/Car Pose Listener2/Subsystem/sensor2vCar ==
  data: x_init output; y_init output; yaw_init output; flag output; poseNew input; poseMsg input
function [x_init,y_init,yaw_init,flag] = sensor2vCar(poseNew, poseMsg)
persistent x0 y0 yaw0 yaw1 x0_init y0_init yaw0_init fStart
if isempty(x0)
    x0=-10; y0=-10; yaw0=0; yaw1=0;   
    x0_init=-10;y0_init=-10;yaw0_init=0;
    fStart=0;
end
if poseNew
    if x0==poseMsg.Pose.Pose.Position.X&&y0==poseMsg.Pose.Pose.Position.Y
        flag=1;
    else
        x0=poseMsg.Pose.Pose.Position.X;
        y0=poseMsg.Pose.Pose.Position.Y;   
        %yaw2=atan2(2*(poseMsg.Pose.Pose.Orientation.Z*poseMsg.Pose.Pose.Orientation.W),1-2*(poseMsg.Pose.Pose.Orientation.Z^2)); 
        eul=quat2eul([poseMsg.Pose.Pose.Orientation.W,poseMsg.Pose.Pose.Orientation.X,poseMsg.Pose.Pose.Orientation.Y,poseMsg.Pose.Pose.Orientation.Z]);
        yaw2=eul(1);
        %对前后角度差使用积分，恢复yaw的连续性
        yaw0=yaw0+angdiff(yaw1,yaw2);
        yaw1=yaw2;
        flag=0;        
        x0_init=x0;
        y0_init=y0;
        yaw0_init=yaw0;
        fStart=1;
    end 
else
    if fStart
        flag=1;
    else
        flag=0;
    end
end

x_init=x0_init;y_init=y0_init;yaw_init=yaw0_init;

== matlab function c6_pfc_rl/Subsystem/Car Pose Listener2/Subsystem/sensor2vCar4 ==
  data: V output; W output; VW_New input; VW_Msg input
function [V,W] = sensor2vCar(VW_New, VW_Msg)
persistent v0 w0
if isempty(v0)
    v0=0; 
    w0=0;    
end
if VW_New
    v0=VW_Msg.Linear.X;
    w0=VW_Msg.Angular.Z;
end

V=v0;
W=-w0;

== matlab function c6_pfc_rl/controller/Ego Car Signal Process1/Signal Process ==
  data: observation output size=[1,9]; obs_flag output; pose1 input; pose2 input; leader_linear_vel input size=1; ego_linear_vel input size=1; ego_omega_vel input size=1; last_ego_omega_vel input
function [observation, obs_flag] = ...
    car2(pose1,pose2,leader_linear_vel, ego_linear_vel, ego_omega_vel, last_ego_omega_vel)


persistent sim_step  yaw_delta lateral_rel_dist

if isempty(sim_step)
    sim_step = 0;
end

if isempty(yaw_delta)
    yaw_delta = 0.0;
end

if isempty(lateral_rel_dist)
    lateral_rel_dist = 0.0;
end

x1=pose1(1);
y1=pose1(2);
yaw1=pose1(3);

x2=pose2(1);
y2=pose2(2);
yaw2=pose2(3);
obs_flag = 1;
observation = zeros(1,9);

if isnan(yaw1)||isnan(yaw2)
    observation = zeros(1,9);
    obs_flag = 0;
    yaw_delta_new = 0.0;
    lateral_rel_dist_new = 0.0;
else
    yaw_delta_new = angdiff(yaw1, yaw2);
    
    [~, lateral_rel_dist_new, longitudinal_rel_dist_new] = heng_zong_dist_calc(x1,y1,x2,y2, yaw1);
    
    observation = get_obs(x1,x2,y1,y2,lateral_rel_dist_new, longitudinal_rel_dist_new, ...
        yaw_delta_new, leader_linear_vel, ego_linear_vel, yaw_delta, lateral_rel_dist); 
end

sim_step = sim_step + 1;
yaw_delta = yaw_delta_new;
lateral_rel_dist = lateral_rel_dist_new;

end

function [rel_dist, heng_dist, zong_dist] = heng_zong_dist_calc(x1,y1,x2,y2, yaw1)

rel_yaw = atan2(y2-y1, x2-x1);

yaw_delta = angdiff(yaw1, rel_yaw);

rel_dist = sqrt(power(x2-x1,2.0)+power(y2-y1,2.0));

heng_dist = rel_dist*sin(yaw_delta);

zong_dist = rel_dist*cos(yaw_delta);

end

function v_ref = get_ref_velocity(leader_linear_vel, ego_linear_vel, longitudinal_rel_dist)
    t_gap = 1.0;
    D_default = 0.3;
    ego_v_set = 0.2;
    d_safe = ego_linear_vel * t_gap + D_default;

    if d_safe > longitudinal_rel_dist
        v_ref = min(leader_linear_vel, ego_v_set);
    else
        v_ref = ego_v_set;
    end
end

function observation = get_obs(x1,x2,y1,y2,lateral_rel_dist_new, longitudinal_rel_dist_new, ...
    yaw_delta_new, leader_linear_vel, ego_linear_vel, yaw_delta, lateral_rel_dist)  
    % 状态空间
    % longitudinal_rel_dist 前车与后车的纵向相对距离
    % lateral_rel_dist 前车与后车的横向相对距离
    % yaw_delta 前车与后车的航向角偏差
    % ego_linear_vel 后车的线速度
    % e_v 后车的参考速度与线速度之差
    % lateral_rel_dist_dot 前车与后车的横向相对距离变化率
    % yaw_delta_dot 前车与后车的航向角偏差变化率

    % 计算前车与后车的相对位置
    x_delta = x1 - x2;
    y_delta = y1 - y2;
    
    % 计算后车的横向偏移距离变化率和相对航向角变化率
    lateral_rel_dist_dot = lateral_rel_dist_new - lateral_rel_dist;
    yaw_delta_dot = yaw_delta_new - yaw_delta;

    % 计算后车的参考速度与线速度之差
    v_ref = get_ref_velocity(leader_linear_vel, ego_linear_vel, longitudinal_rel_dist_new);
    e_v = v_ref - ego_linear_vel;

    observation = [x_delta/2.0, y_delta/2.0, longitudinal_rel_dist_new/2.0, e_v/0.5, ego_linear_vel/0.5, ...
        lateral_rel_dist_new/2.0, lateral_rel_dist_dot/2.0, yaw_delta_new/pi, yaw_delta_dot/pi];
end

function flag = EnvisDone(rel_dist, lateral_rel_dist, longitudinal_rel_dist)
    flag = 0;
    avoid_dist = 0.14;

    max_lateral_rel_dist= 0.45;
    min_longitudinal_rel_dist = -0.5;

    if rel_dist <= avoid_dist
        flag = 1;
    end

    if longitudinal_rel_dist <= min_longitudinal_rel_dist
        flag = 1;
    end
    
    if abs(lateral_rel_dist) >= max_lateral_rel_dist
        flag = 1;
    end
end

function reward = reward_calc(e_v, lateral_rel_dist, ego_linear_vel, ego_omega_vel, last_ego_omega_vel, isDone, sim_step)
    F_t = 0.0;
    M_t = 0.0;
    H_t = 0.0;
    delta_omega = 0.0;
    
    e_v_square = e_v * e_v;
    lateral_rel_dist_square = lateral_rel_dist * lateral_rel_dist;

    if isDone==1
        F_t = 1.0;
    end

    if e_v_square < 1.0
        M_t = 1.0;
    end

    if lateral_rel_dist_square<0.01
        H_t = 1.0;
    end

    if sim_step >= 2
        delta_omega = ego_omega_vel - last_ego_omega_vel;
    end

    reward = -0.1*e_v_square - 0.1*ego_linear_vel*ego_linear_vel -0.1*lateral_rel_dist_square ...
         - 0.5*ego_omega_vel*ego_omega_vel -0.4*delta_omega*delta_omega - 10.0*F_t + M_t + + 2.0*H_t;

end

== matlab function c6_pfc_rl/controller/Subsystem1/Adjust Velocities to Avoid Obstacles/Path Following/Compute Angular Velocity ==
  data: steeringDir input; w output; wMax input
function w = exampleHelperComputeAngularVelocity(steeringDir, wMax)
%EXAMPLEHELPERCOMPUTEANGULARVELOCITY Compute angular velocity
%   W = exampleHelperComputeAngularVelocity(STEERINGDIR)
%   returns the angular velocity W for a differential drive robot in radians
%   per second for a given steering direction STEERINGDIR in the robot's
%   coordinate frame in radians.
%
%   W = exampleHelperComputeAngularVelocity(STEERINGDIR, WMAX)
%   returns the angular velocity W for a differential drive robot in radians
%   per second for a given steering direction STEERINGDIR in the robot's
%   coordinate frame in radians and maximum angular velocity WMAX in
%   radians per second. The output angular velocity is saturated based on
%   the WMAX.
%
%   Example:
%       
%       w = exampleHelperComputeAngularVelocity(0.2, 1);

% Copyright 2015 The MathWorks, Inc.

%#codegen
%#ok<*EMCA>

% Allow variable input arguments
if nargin == 1   
    wMax = inf;
end

validateattributes(steeringDir, {'double'},{'real'},...
    'exampleHelperComputeAngularVelocity', 'STEERINGDIR', 1);
validateattributes(wMax, {'double'},{'real', 'positive'},...
    'exampleHelperComputeAngularVelocity', 'WMAX', 2);

% Computing in robot's coordinate frame
curPose = [0 0 0];

% The following computation is similar to robotics.PurePursuit
lookaheadPoint = [cos(steeringDir), sin(steeringDir)];
slope = atan2((lookaheadPoint(2) - curPose(2)), ...
    (lookaheadPoint(1) - curPose(1)));
alpha = angdiff(curPose(3), slope);

% Angular velocity command for a differential drive robot is
% equal to the desired curvature to be followed by the robot.

w = (2*sin(alpha));

% Pick a constant rotation when robot is facing in the opposite
% direction of the path
if abs(abs(alpha) - pi) < 1e-12
    w = sign(w)*1;
end

if abs(w) > wMax
    w = sign(w)*wMax;
end

end

== matlab function c6_pfc_rl/controller/Subsystem1/Compute Velocity and Heading for Path following/ Extract Goal ==
  data: Waypoints input; Goal output
function Goal = extractGoal(Waypoints)
%#codegen
b = isnan(Waypoints);
[rows,~] = find(b);
ridx = setdiff(1:size(Waypoints,1), sort(rows));
Goal = [Waypoints(ridx(end), 1) Waypoints(ridx(end), 2)];

== matlab function c6_pfc_rl/controller/MATLAB Function1 ==
  settings: updateMethod=DISCRETE
  data: obs input double size=9; pose2 input; action output double size=[1,2]; obs_flag input
function action = one_car_pfc(obs, pose2, obs_flag)

longitudinal_rel_dist = obs(3);
lateral_rel_dist = obs(6);

if longitudinal_rel_dist > -0.25 && abs(lateral_rel_dist) <=0.225 && longitudinal_rel_dist < 0
    action = double(PFC_Policy(obs));
else
    action = simple_pfc(obs(1), obs(2), pose2(3));
end

if obs_flag==0
    action = [0.0, 0.0];
end

end

function action = simple_pfc(x_delta, y_delta, yaw2)
    kk = -1.0;

    new_theta_cmd = atan2(y_delta, x_delta);
    
    delta_theta = angdiff(yaw2, new_theta_cmd);

    angular_speed = kk * delta_theta;

    new_omega_cmd = angular_speed;

    action = [0.225, new_omega_cmd];

end
